simulink model "gm_VSD_6ph_30deg_HDL"  (R2021a)
settings: Solver=FixedStepDiscrete  StartTime=0.0  StopTime=1/f  RelTol=1e-3
undefined symbols (not defined in the file or in its folder): t_ADC
libraries: fl_lib x7, nesl_utility x7, ee_lib x2, simulink x1
settings Model: Creator=micha  LastModifiedBy=micha
settings SolverCC: AlgebraicLoopSolver=TrustRegion
settings DataIOCC: LimitDataPoints=on  SaveOutput=off  SaveTime=off
settings OptimizationCC: BlockReduction=off  ConditionallyExecuteInputs=off  DefaultParameterBehavior=Inlined  LifeSpan=inf
settings DebuggingCC: AlgebraicLoopMsg=error  InheritedTsInSrcMsg=none  SingleTaskRateTransMsg=error  AllowSymbolicDim=off  StrictBusMsg=ErrorOnBusTreatedAsVector  SFUnexpectedBacktrackingDiag=warning  SFNoUnconditionalDefaultTransitionDiag=warning  SFExecutionAtInitializationDiag=none  SFMachineParentedDataDiag=warning  ArithmeticOperatorsInVariantConditions=warning
settings HardwareCC: ProdBitPerPointer=32  ProdBitPerSizeT=32  ProdBitPerPtrDiffT=32  ProdLargestAtomicFloat=None  ProdIntDivRoundTo=Undefined  ProdEndianess=Unspecified  ProdWordSize=32  ProdHWDeviceType=ASIC/FPGA->ASIC/FPGA  ProdEqTarget=off
settings SFSimCC: SimUseLocalCustomCode=off  CustomCodeUndefinedFunction=UseInterfaceOnly
settings RTWCC: RTWUseLocalCustomCode=off
settings CodeAppCC: StateflowObjectComments=on
settings GRTTargetCC: TargetLangStandard=C89/C90 (ANSI)
settings ConfigComp: CovScope=ReferencedModels  CovMetricSettings=dw  CovSaveCumulativeToWorkspaceVar=on  CovSaveSingleToWorkspaceVar=on  CovExternalEMLEnable=off  CovSFcnEnable=off

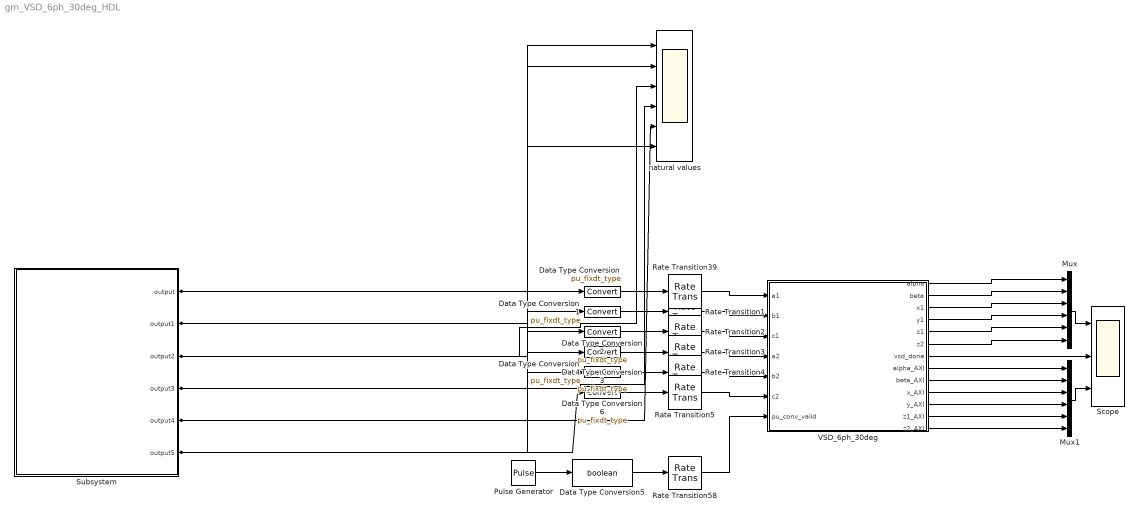
== system gm_VSD_6ph_30deg_HDL ==
  Data Type Conversion{,1..4,6} (6 alike) : DataTypeConversion  OutDataTypeStr=pu_fixdt_type
  Data Type Conversion5 : DataTypeConversion  OutDataTypeStr=boolean
  Mux : Mux  Inputs=6
  Mux1 : Mux  Inputs=6
  Pulse Generator : DiscretePulseGenerator  PulseType=Time based  Period=t_ADC  PulseWidth=5
  Rate Transition{1..5,39,58} (7 alike) : RateTransition  OutPortSampleTime=ts
  Scope : Scope  NumInputPorts=3
  Subsystem : Subsystem
  VSD_6ph_30deg : Subsystem  TreatAsAtomicUnit=on
  natural values : Scope  NumInputPorts=6
  wires:
  Mux1/1 -> Scope/3
  VSD_6ph_30deg/13(z2_AXI) -> Mux1/6
  VSD_6ph_30deg/12(z1_AXI) -> Mux1/5
  VSD_6ph_30deg/11(y_AXI) -> Mux1/4
  VSD_6ph_30deg/10(x_AXI) -> Mux1/3
  VSD_6ph_30deg/9(beta_AXI) -> Mux1/2
  VSD_6ph_30deg/8(alpha_AXI) -> Mux1/1
  Subsystem/1(output) -> Data Type Conversion/1, natural values/1
  Subsystem/4(output3) -> natural values/4, Data Type Conversion3/1
  Subsystem/5(output4) -> natural values/5, Data Type Conversion4/1
  Subsystem/2(output1) -> Data Type Conversion1/1, natural values/2
  Subsystem/3(output2) -> natural values/3, Data Type Conversion2/1
  Subsystem/6(output5) -> Data Type Conversion6/1, natural values/6
  Data Type Conversion6/1 -> Rate Transition5/1
  Data Type Conversion4/1 -> Rate Transition4/1
  Data Type Conversion3/1 -> Rate Transition3/1
  Data Type Conversion2/1 -> Rate Transition2/1
  Data Type Conversion1/1 -> Rate Transition1/1
  Data Type Conversion/1 -> Rate Transition39/1
  Rate Transition4/1 -> VSD_6ph_30deg/5(b2)
  Rate Transition3/1 -> VSD_6ph_30deg/4(a2)
  Rate Transition2/1 -> VSD_6ph_30deg/3(c1)
  Rate Transition39/1 -> VSD_6ph_30deg/1(a1)
  Rate Transition1/1 -> VSD_6ph_30deg/2(b1)
  Mux/1 -> Scope/1
  VSD_6ph_30deg/7(vsd_done) -> Scope/2
  VSD_6ph_30deg/6(z2) -> Mux/6
  VSD_6ph_30deg/5(z1) -> Mux/5
  VSD_6ph_30deg/4(y1) -> Mux/4
  VSD_6ph_30deg/3(x1) -> Mux/3
  VSD_6ph_30deg/2(beta) -> Mux/2
  VSD_6ph_30deg/1(alpha) -> Mux/1
  Rate Transition5/1 -> VSD_6ph_30deg/6(c2)
  Rate Transition58/1 -> VSD_6ph_30deg/7(pu_conv_valid)
  Data Type Conversion5/1 -> Rate Transition58/1
  Pulse Generator/1 -> Data Type Conversion5/1

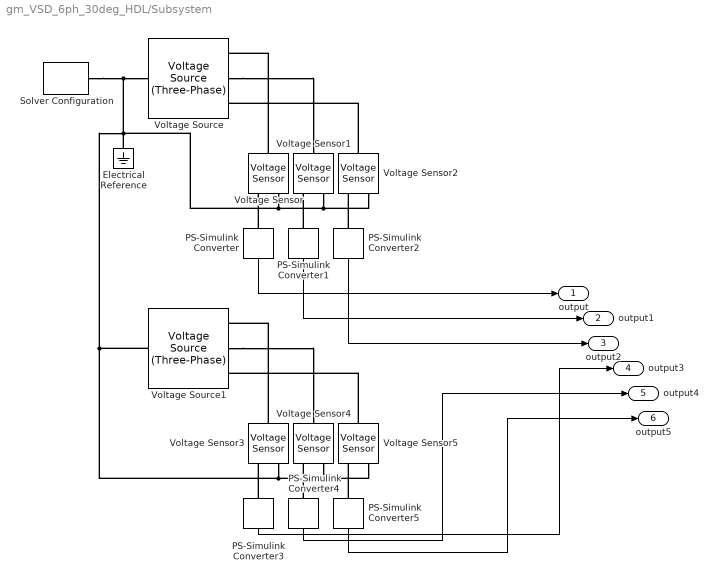
== system gm_VSD_6ph_30deg_HDL/Subsystem ==
  Electrical Reference : fl_lib/Electrical/Electrical Elements/Electrical Reference
  PS-Simulink Converter{,1..5} (6 alike) : nesl_utility/PS-Simulink Converter  PhysicalDomain=network_engine_domain  SubClassName=ps_output  LeftPortType=input  RightPortType=output  PseudoPeriodic=off  Frequencies=[]  Unit=1  AffineConversion=off
  Solver Configuration : nesl_utility/Solver Configuration  PhysicalDomain=network_engine_domain  SubClassName=solver  LeftPortType=input  RightPortType=generic  Tones=[]  Harmonics=[]  SimulateNoise=off  Profile=off  UseLocalSampling=off  EnableSwitchedLinearOptims=on  FrequencyDomain=off  UseCCode=off  RelTol=0.001  AbsTol=1e-06  MinStep=1e-09  ToWorkspace=off  RevertToSquareIcSolve=off  NumHomotopyIterations=100  PhasorMode=off  PhasorModeNumHarmonics=1  DoDC=off  ResidualTolerance=1e-09  UseLocalSolver=on  LocalSolverChoice=NE_BACKWARD_EULER_ADVANCER  LocalSolverSampleTime=1e-6  DoFixedCost=on  MaxNonlinIter=3  MaxModeIter=2  ComputeImpulses=off  ImpulseIterations=2  LinearAlgebra=Sparse  EquationFormulation=NE_TIME_EF  DelaysMemoryBudget=1024  AutomaticFiltering=on  FilteringTimeConstant=0.001  PartitionStorageMethod=AS_NEEDED  PartitionMemoryBudget=1024  PartitionMethod=FAST
  Voltage Sensor{,1..5} (6 alike) : fl_lib/Electrical/Electrical Sensors/Voltage Sensor
  Voltage Source : ee_lib/Sources/Voltage Source (Three-Phase)  vline_rms=1*sqrt(3)/sqrt(2) V  shift=0 deg  freq=f Hz  impedance_option=1  SShortCircuit=1e6 V*A  XR=15  R=0.01 Ohm  L=3.97e-4 H  G_parasitic=0 1/Ohm  harmonic_option=1  harmonic_orders=Harmonic_Orders  harmonic_ratios=Harmonic_Amplitudes  I_specify=off  I_priority=None  I=[ 0 0 0 ] A  I_nominal_specify=off  I_nominal_unit=A  I_nominal_value=1
      settings: SourceProductBaseCode=PS  InternalSimscapePortConfiguration="{\"Bottom\":[],\"Left\":[{\"id\":\"n\",\"label\":\"n\",\"type\":\"foundation.electrical.electrical\"}],\"Right\":[{\"id\":\"a\",\"label\":\"a\",\"type\":\"foundation.electrical.electrical\"},{\"id\":\"b\",\"label\":\"b\",\"type\":\"foundation.electrical.electrical\"},{\"id\":\"c\",\"label\":\"c\",\"type\":\"foundation.electrical.electrical\"}],\"Top\":[]}"
  Voltage Source1 : ee_lib/Sources/Voltage Source (Three-Phase)  vline_rms=1*sqrt(3)/sqrt(2) V  shift=-30 deg  freq=f Hz  impedance_option=1  SShortCircuit=1e6 V*A  XR=15  R=0.01 Ohm  L=3.97e-4 H  G_parasitic=0 1/Ohm  harmonic_option=1  harmonic_orders=Harmonic_Orders  harmonic_ratios=Harmonic_Amplitudes  I_specify=off  I_priority=None  I=[ 0 0 0 ] A  I_nominal_specify=off  I_nominal_unit=A  I_nominal_value=1
      settings: SourceProductBaseCode=PS  InternalSimscapePortConfiguration="{\"Bottom\":[],\"Left\":[{\"id\":\"n\",\"label\":\"n\",\"type\":\"foundation.electrical.electrical\"}],\"Right\":[{\"id\":\"a\",\"label\":\"a\",\"type\":\"foundation.electrical.electrical\"},{\"id\":\"b\",\"label\":\"b\",\"type\":\"foundation.electrical.electrical\"},{\"id\":\"c\",\"label\":\"c\",\"type\":\"foundation.electrical.electrical\"}],\"Top\":[]}"
  output : Outport
  output1 : Outport  Port=2
  output2 : Outport  Port=3
  output3 : Outport  Port=4
  output4 : Outport  Port=5
  output5 : Outport  Port=6
  wires:
  PS-Simulink Converter2/1 -> output2/1
  PS-Simulink Converter5/1 -> output5/1
  PS-Simulink Converter1/1 -> output1/1
  PS-Simulink Converter4/1 -> output4/1
  PS-Simulink Converter3/1 -> output3/1
  PS-Simulink Converter/1 -> output/1
  connections:
  Voltage Source/RConn2 -- Voltage Sensor1/LConn1
  Voltage Sensor/LConn1 -- Voltage Source/RConn1
  PS-Simulink Converter3/LConn1 -- Voltage Sensor3/RConn1
  PS-Simulink Converter2/LConn1 -- Voltage Sensor2/RConn1
  Voltage Sensor2/LConn1 -- Voltage Source/RConn3
  PS-Simulink Converter4/LConn1 -- Voltage Sensor4/RConn1
  Voltage Sensor5/LConn1 -- Voltage Source1/RConn3
  Voltage Source1/RConn2 -- Voltage Sensor4/LConn1
  PS-Simulink Converter/LConn1 -- Voltage Sensor/RConn1
  Voltage Sensor3/LConn1 -- Voltage Source1/RConn1
  PS-Simulink Converter1/LConn1 -- Voltage Sensor1/RConn1
  PS-Simulink Converter5/LConn1 -- Voltage Sensor5/RConn1
  Voltage Sensor4/RConn2 -- Voltage Sensor3/RConn2 -- Voltage Source1/LConn1 -- Electrical Reference/LConn1 -- Voltage Sensor/RConn2 -- Voltage Sensor1/RConn2 -- Voltage Sensor2/RConn2 -- Voltage Source/LConn1 -- Solver Configuration/RConn1 -- Voltage Sensor5/RConn2

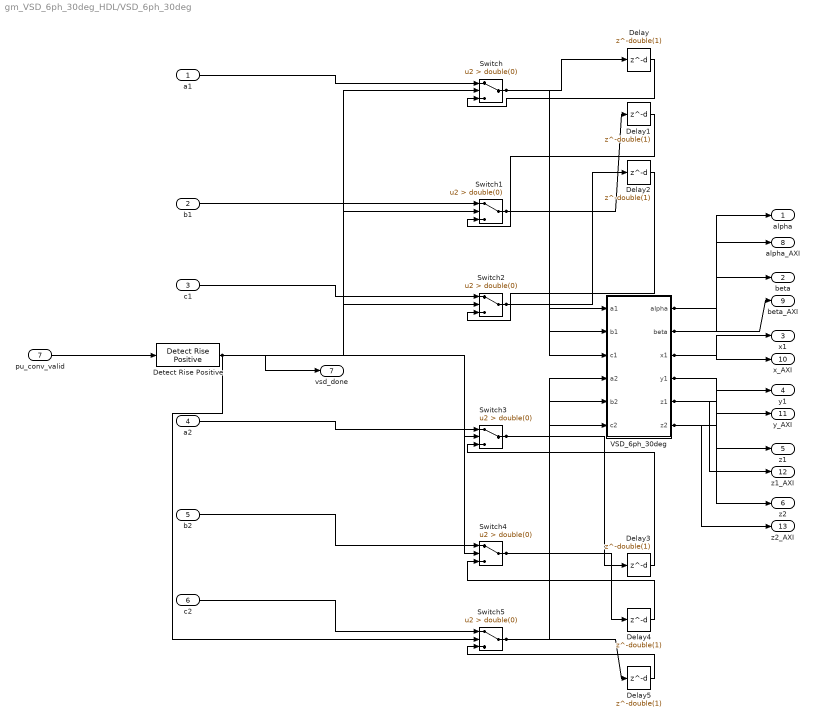
== system gm_VSD_6ph_30deg_HDL/VSD_6ph_30deg ==
  a1 : Inport  OutDataTypeStr=fixdt(1, 18, 15)  PortDimensions=1  SampleTime=1e-08
  b1 : Inport  Port=2  OutDataTypeStr=fixdt(1, 18, 15)  PortDimensions=1  SampleTime=1e-08
  c1 : Inport  Port=3  OutDataTypeStr=fixdt(1, 18, 15)  PortDimensions=1  SampleTime=1e-08
  a2 : Inport  Port=4  OutDataTypeStr=fixdt(1, 18, 15)  PortDimensions=1  SampleTime=1e-08
  b2 : Inport  Port=5  OutDataTypeStr=fixdt(1, 18, 15)  PortDimensions=1  SampleTime=1e-08
  c2 : Inport  Port=6  OutDataTypeStr=fixdt(1, 18, 15)  PortDimensions=1  SampleTime=1e-08
  pu_conv_valid : Inport  Port=7  OutDataTypeStr=boolean  PortDimensions=1  SampleTime=1e-08
  Delay{,1..5} (6 alike) : Delay  DelayLength=double(1)  InitialCondition=0  SampleTime=1e-08
  Detect Rise Positive : simulink/Logic and Bit Operations/Detect Rise Positive  vinit=0  OutDataTypeStr=boolean
  Switch{,1..5} (6 alike) : Switch  Criteria=u2 > Threshold  Threshold=double(0)  OutDataTypeStr=fixdt(1, 18, 15)  SampleTime=1e-08
  VSD_6ph_30deg : Subsystem
  alpha : Outport  OutDataTypeStr=fixdt(1,18,11)  SampleTime=1e-08  VectorParamsAs1DForOutWhenUnconnected=off
  beta : Outport  Port=2  OutDataTypeStr=fixdt(1,18,11)  SampleTime=1e-08  VectorParamsAs1DForOutWhenUnconnected=off
  x1 : Outport  Port=3  OutDataTypeStr=fixdt(1,18,11)  SampleTime=1e-08  VectorParamsAs1DForOutWhenUnconnected=off
  y1 : Outport  Port=4  OutDataTypeStr=fixdt(1,18,11)  SampleTime=1e-08  VectorParamsAs1DForOutWhenUnconnected=off
  z1 : Outport  Port=5  OutDataTypeStr=fixdt(1,18,11)  SampleTime=1e-08  VectorParamsAs1DForOutWhenUnconnected=off
  z2 : Outport  Port=6  OutDataTypeStr=fixdt(1,18,11)  SampleTime=1e-08  VectorParamsAs1DForOutWhenUnconnected=off
  vsd_done : Outport  Port=7  SampleTime=1e-08  VectorParamsAs1DForOutWhenUnconnected=off
  alpha_AXI : Outport  Port=8  OutDataTypeStr=fixdt(1,18,11)  SampleTime=1e-08  VectorParamsAs1DForOutWhenUnconnected=off
  beta_AXI : Outport  Port=9  OutDataTypeStr=fixdt(1,18,11)  SampleTime=1e-08  VectorParamsAs1DForOutWhenUnconnected=off
  x_AXI : Outport  Port=10  OutDataTypeStr=fixdt(1,18,11)  SampleTime=1e-08  VectorParamsAs1DForOutWhenUnconnected=off
  y_AXI : Outport  Port=11  OutDataTypeStr=fixdt(1,18,11)  SampleTime=1e-08  VectorParamsAs1DForOutWhenUnconnected=off
  z1_AXI : Outport  Port=12  OutDataTypeStr=fixdt(1,18,11)  SampleTime=1e-08  VectorParamsAs1DForOutWhenUnconnected=off
  z2_AXI : Outport  Port=13  OutDataTypeStr=fixdt(1,18,11)  SampleTime=1e-08  VectorParamsAs1DForOutWhenUnconnected=off
  wires:
  a1/1 -> Switch/1
  b1/1 -> Switch1/1
  c1/1 -> Switch2/1
  a2/1 -> Switch3/1
  b2/1 -> Switch4/1
  c2/1 -> Switch5/1
  pu_conv_valid/1 -> Detect Rise Positive/1
  Delay/1 -> Switch/3
  Delay1/1 -> Switch1/3
  Delay2/1 -> Switch2/3
  Delay3/1 -> Switch3/3
  Delay4/1 -> Switch4/3
  Delay5/1 -> Switch5/3
  Detect Rise Positive/1 -> Switch5/2, Switch4/2, Switch3/2, Switch2/2, Switch1/2, Switch/2, vsd_done/1
  Switch/1 -> Delay/1, VSD_6ph_30deg/1(a1)
  Switch1/1 -> Delay1/1, VSD_6ph_30deg/2(b1)
  Switch2/1 -> Delay2/1, VSD_6ph_30deg/3(c1)
  Switch3/1 -> Delay3/1, VSD_6ph_30deg/4(a2)
  Switch4/1 -> Delay4/1, VSD_6ph_30deg/5(b2)
  Switch5/1 -> Delay5/1, VSD_6ph_30deg/6(c2)
  VSD_6ph_30deg/1(alpha) -> alpha_AXI/1, alpha/1
  VSD_6ph_30deg/2(beta) -> beta_AXI/1, beta/1
  VSD_6ph_30deg/3(x1) -> x_AXI/1, x1/1
  VSD_6ph_30deg/4(y1) -> y_AXI/1, y1/1
  VSD_6ph_30deg/5(z1) -> z1_AXI/1, z1/1
  VSD_6ph_30deg/6(z2) -> z2_AXI/1, z2/1

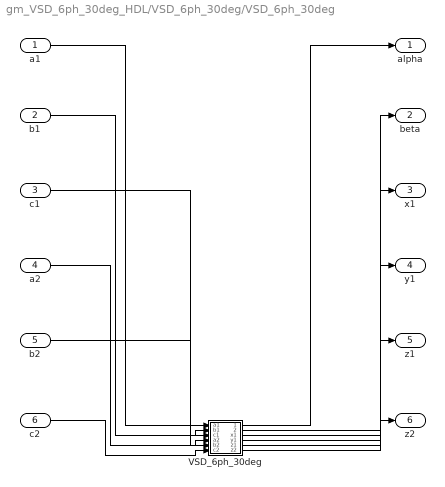
== system gm_VSD_6ph_30deg_HDL/VSD_6ph_30deg/VSD_6ph_30deg ==
  a1 : Inport  OutDataTypeStr=fixdt(1, 18, 15)  PortDimensions=1  SampleTime=1e-08
  b1 : Inport  Port=2  OutDataTypeStr=fixdt(1, 18, 15)  PortDimensions=1  SampleTime=1e-08
  c1 : Inport  Port=3  OutDataTypeStr=fixdt(1, 18, 15)  PortDimensions=1  SampleTime=1e-08
  a2 : Inport  Port=4  OutDataTypeStr=fixdt(1, 18, 15)  PortDimensions=1  SampleTime=1e-08
  b2 : Inport  Port=5  OutDataTypeStr=fixdt(1, 18, 15)  PortDimensions=1  SampleTime=1e-08
  c2 : Inport  Port=6  OutDataTypeStr=fixdt(1, 18, 15)  PortDimensions=1  SampleTime=1e-08
  VSD_6ph_30deg : MATLAB Function  TreatAsAtomicUnit=on
  alpha : Outport  SampleTime=1e-08
  beta : Outport  Port=2  SampleTime=1e-08
  x1 : Outport  Port=3  SampleTime=1e-08
  y1 : Outport  Port=4  SampleTime=1e-08
  z1 : Outport  Port=5  SampleTime=1e-08
  z2 : Outport  Port=6  SampleTime=1e-08
  wires:
  a1/1 -> VSD_6ph_30deg/1(a1)
  b1/1 -> VSD_6ph_30deg/2(b1)
  c1/1 -> VSD_6ph_30deg/3(c1)
  a2/1 -> VSD_6ph_30deg/4(a2)
  b2/1 -> VSD_6ph_30deg/5(b2)
  c2/1 -> VSD_6ph_30deg/6(c2)
  VSD_6ph_30deg/1(alpha) -> alpha/1
  VSD_6ph_30deg/2(beta) -> beta/1
  VSD_6ph_30deg/3(x1) -> x1/1
  VSD_6ph_30deg/4(y1) -> y1/1
  VSD_6ph_30deg/5(z1) -> z1/1
  VSD_6ph_30deg/6(z2) -> z2/1

== matlab function gm_VSD_6ph_30deg_HDL/VSD_6ph_30deg/VSD_6ph_30deg/VSD_6ph_30deg ==
  data: a1 input; alpha output; b1 input; c1 input; a2 input; b2 input; c2 input; beta output; x1 output; y1 output; z1 output; z2 output
function [alpha,beta,x1,y1,z1,z2] = fcn(a1,b1,c1,a2,b2,c2)


A = [fi(0,1,18,11) fi(0,1,18,11) fi(0,1,18,11) fi(0,1,18,11) fi(0,1,18,11) fi(0,1,18,11)]';

A =    2/6*[1    -0.5        -0.5        sqrt(3)/2   -sqrt(3)/2  0 ;
           0    sqrt(3)/2   -sqrt(3)/2  0.5         0.5         -1;
           1    -0.5        -0.5        -sqrt(3)/2  sqrt(3)/2   0 ;
           0    -sqrt(3)/2  sqrt(3)/2   0.5         0.5         -1;
           0.5   0.5          0.5          0           0           0 ;
           0    0           0           0.5          0.5          0.5] * [a1 b1 c1 a2 b2 c2]';

alpha = fi(A(1),1,18,11);
beta = fi(A(2),1,18,11);
x1 = fi(A(3),1,18,11);
y1 = fi(A(4),1,18,11);
z1 = fi(A(5),1,18,11);
z2 = fi(A(6),1,18,11);
